simulink subsystem "Inverter_and_Motor"  (R2024a)
settings: Solver=VariableStepAuto  StartTime=0.0  StopTime=10.0  RelTol=1e-3
values from neighbouring files (symbols this model uses):
  PI_params_SI = mcb.internal.SetControllerParameters(pmsm,inverter,SI_System,T_pwm,Ts,Ts_speed)    [mchp_pmsm_foc_smo_dsPIC33_data.m]
  Ts = T_pwm    (= 5e-05)    [mchp_pmsm_foc_smo_dsPIC33_data.m]
undefined symbols (not defined in the file or in its folder): inverter, pmsm
libraries: mcbplantlib x1, mcbcontrolslib x1, autolibpmsmexterior x1
settings Model: Creator=I50990  LastModifiedBy=I67977
settings RTWCC: GPUComputeCapability=3.5

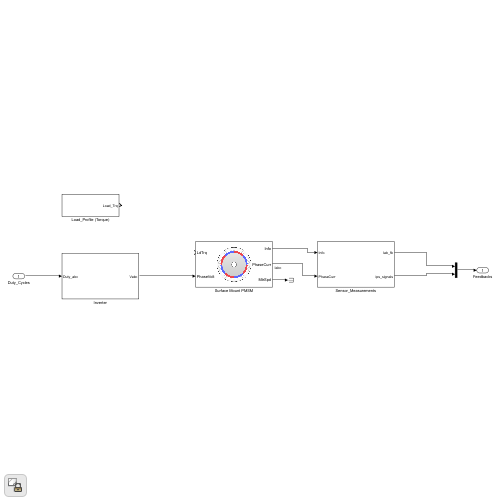
[thumbnail: Simulink's stored preview of the top-level diagram]
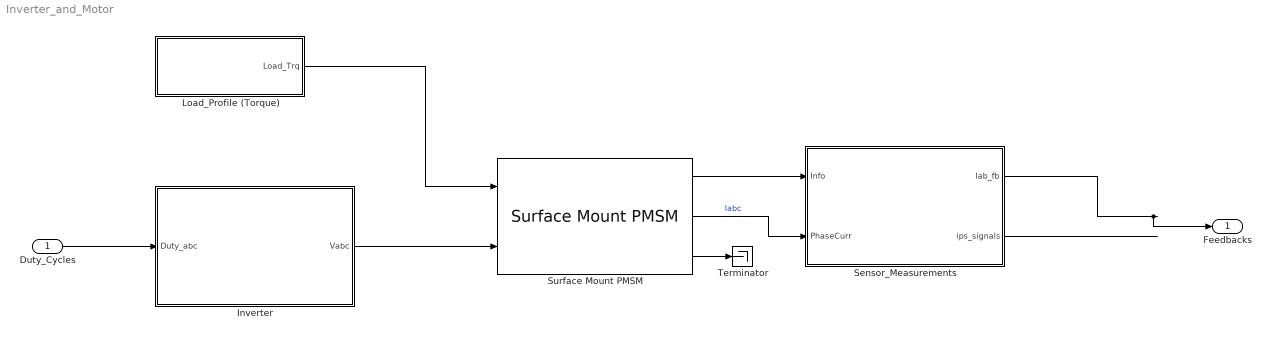
== system Inverter_and_Motor ==
  Duty_Cycles : Inport
  Inverter : Subsystem
  Load_Profile (Torque) : Subsystem
  Sensor_Measurements : Subsystem
  Surface Mount PMSM : autolibpmsmexterior/Surface Mount PMSM  port_config=Torque  sim_type=Discrete  Ts=Ts  P=pmsm.p  Rs=pmsm.Rs + inverter.R_board  Ldq_=pmsm.Ld  KConstText=Permanent flux linkage constant (lambda_pm):  lambda_pm=pmsm.FluxPM  Ke=159.9771  Kt=1.323  mechanical=[pmsm.J, pmsm.B, 0]  idq0=[0 0]  theta_init=0  omega_init=0  KConst=pmsm.FluxPM  lambda_pm_calc=pmsm.FluxPM  RefBlkName='autolibpmsmexterior/Surface Mount PMSM'  aMode=5  Ldq="[0.0002      0.0002]"
  Terminator : Terminator
  Feedbacks : Outport  VectorParamsAs1DForOutWhenUnconnected=off
  wires:
  Surface Mount PMSM/1 -> Sensor_Measurements/1(Info)
  Surface Mount PMSM/2 -> Sensor_Measurements/2(PhaseCurr)  "Iabc"
  Surface Mount PMSM/3 -> Terminator/1
  Sensor_Measurements/2(ips_signals) -> ?
  Duty_Cycles/1 -> Inverter/1(Duty_abc)
  Inverter/1(Vabc) -> Surface Mount PMSM/2
  Sensor_Measurements/1(Iab_fb) -> Feedbacks/1
  Load_Profile (Torque)/1(Load_Trq) -> Surface Mount PMSM/1

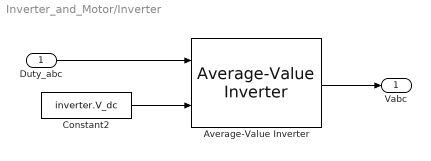
== system Inverter_and_Motor/Inverter ==
  Duty_abc : Inport
  Average-Value Inverter : mcbplantlib/Average-Value Inverter
  Constant2 : Constant  Value=inverter.V_dc  OutDataTypeStr=single  SampleTime=-1
  Vabc : Outport  VectorParamsAs1DForOutWhenUnconnected=off
  wires:
  Constant2/1 -> Average-Value Inverter/2
  Duty_abc/1 -> Average-Value Inverter/1
  Average-Value Inverter/1 -> Vabc/1

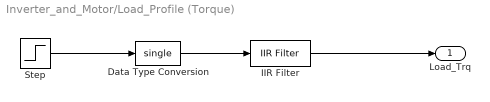
== system Inverter_and_Motor/Load_Profile (Torque) ==
  Data Type Conversion : DataTypeConversion  OutDataTypeStr=single  SaturateOnIntegerOverflow=off  RndMeth=Floor
  IIR Filter : mcbcontrolslib/IIR Filter  VariantControl=Low Pass Filter  VariantSelect=Low-pass  FilterConstantInputType=Specify via dialog  Filter_constant=0.01  advancedSettings=off  Ts=50e-6  cutOff_freq=32.1525
  Step : Step  Time=6  Before=0.00 * pmsm.T_rated  After=0.015 * pmsm.T_rated  SampleTime=Ts
  Load_Trq : Outport  VectorParamsAs1DForOutWhenUnconnected=off
  wires:
  Step/1 -> Data Type Conversion/1
  Data Type Conversion/1 -> IIR Filter/1
  IIR Filter/1 -> Load_Trq/1

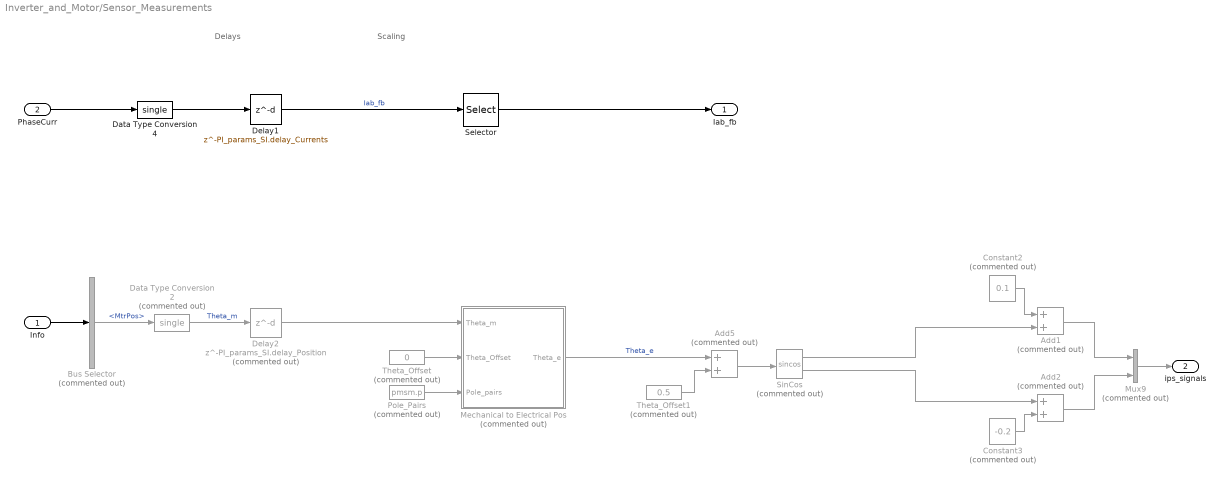
== system Inverter_and_Motor/Sensor_Measurements ==
  note: Delays
  note: Scaling
  Info : Inport
  PhaseCurr : Inport  Port=2
  Add1 : Sum  Commented=on
  Add2 : Sum  Commented=on
  Add5 : Sum  Commented=on
  Bus Selector : BusSelector  Commented=on  OutputSignals=MtrPos
  Constant2 : Constant  Commented=on  Value=0.1  OutDataTypeStr=single  SampleTime=Ts
  Constant3 : Constant  Commented=on  Value=-0.2  OutDataTypeStr=single  SampleTime=Ts
  Data Type Conversion2 : DataTypeConversion  Commented=on  OutDataTypeStr=single  RndMeth=Simplest  SaturateOnIntegerOverflow=off
  Data Type Conversion4 : DataTypeConversion  OutDataTypeStr=single  RndMeth=Simplest  SaturateOnIntegerOverflow=off
  Delay1 : Delay  DelayLength=PI_params_SI.delay_Currents
  Delay2 : Delay  Commented=on  DelayLength=PI_params_SI.delay_Position
  Mechanical to Electrical Pos : Subsystem  Commented=on
  Mux9 : Mux  Commented=on  Inputs=2
  Pole_Pairs : Constant  Commented=on  Value=pmsm.p  OutDataTypeStr=dataType  SampleTime=Ts
  Selector : Selector  InputPortWidth=3  IndexOptions=Index vector (dialog)  Indices=[1 2]  OutputSizes=1
  SinCos : Trigonometry  Commented=on  Operator=sincos
  Theta_Offset : Constant  Commented=on  Value=0  OutDataTypeStr=dataType  SampleTime=Ts
  Theta_Offset1 : Constant  Commented=on  Value=0.5  OutDataTypeStr=dataType  SampleTime=Ts
  Iab_fb : Outport  VectorParamsAs1DForOutWhenUnconnected=off
  ips_signals : Outport  Port=2  VectorParamsAs1DForOutWhenUnconnected=off
  wires:
  Add5/1 -> SinCos/1
  Theta_Offset1/1 -> Add5/2
  Constant2/1 -> Add1/1
  Constant3/1 -> Add2/2
  Mechanical to Electrical Pos/1(Theta_e) -> Add5/1  "Theta_e"
  Theta_Offset/1 -> Mechanical to Electrical Pos/2(Theta_Offset)
  Pole_Pairs/1 -> Mechanical to Electrical Pos/3(Pole_pairs)
  SinCos/2 -> Add2/1
  SinCos/1 -> Add1/2
  Add1/1 -> Mux9/1
  Mux9/1 -> ips_signals/1
  Add2/1 -> Mux9/2
  Delay2/1 -> Mechanical to Electrical Pos/1(Theta_m)
  Data Type Conversion2/1 -> Delay2/1  "Theta_m"
  Bus Selector/1 -> Data Type Conversion2/1  "<MtrPos>"
  Info/1 -> Bus Selector/1
  PhaseCurr/1 -> Data Type Conversion4/1
  Data Type Conversion4/1 -> Delay1/1
  Delay1/1 -> Selector/1  "Iab_fb"
  Selector/1 -> Iab_fb/1

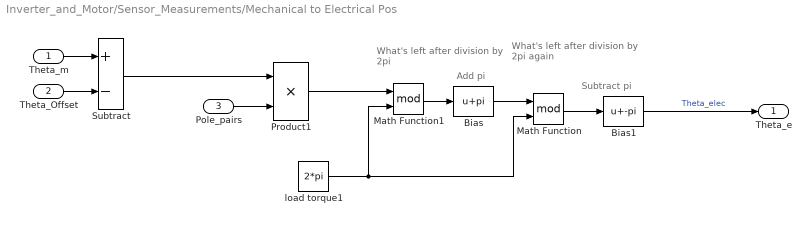
== system Inverter_and_Motor/Sensor_Measurements/Mechanical to Electrical Pos ==
  note: Subtract pi
  note: What's left after
      | division by 2pi
      | again
  note: What's left after
      | division by 2pi
  note: Add pi
  Theta_m : Inport
  Theta_Offset : Inport  Port=2
  Pole_pairs : Inport  Port=3
  Bias : Bias  Bias=pi  SaturateOnIntegerOverflow=off
  Bias1 : Bias  Bias=-pi  SaturateOnIntegerOverflow=off
  Math Function : Math  Operator=mod  SignedPower=on
  Math Function1 : Math  Operator=mod  SignedPower=on
  Product1 : Product  RndMeth=Simplest  OutDataTypeStr=Inherit: Same as first input
  Subtract : Sum  Inputs=+-
  load torque1 : Constant  Value=2*pi  OutDataTypeStr=single  SampleTime=Ts
  Theta_e : Outport
  wires:
  Theta_Offset/1 -> Subtract/2
  Subtract/1 -> Product1/1
  Theta_m/1 -> Subtract/1
  Product1/1 -> Math Function1/1
  load torque1/1 -> Math Function/2, Math Function1/2
  Bias1/1 -> Theta_e/1  "Theta_elec"
  Math Function1/1 -> Bias/1
  Bias/1 -> Math Function/1
  Pole_pairs/1 -> Product1/2
  Math Function/1 -> Bias1/1
